simulink model "intrari_necunoscute"  (R2022b)
settings: Solver=VariableStepAuto  StartTime=0.0  StopTime=100  RelTol=1e-3
values from neighbouring files (symbols this model uses):
  A = [0 0 1 0 ... (first row only)    [cmsd_script.m]
  Ae = [A,E;zeros(1,5)]    [cmsd_script.m]
  B = [0,0 ... (first row only)    [cmsd_script.m]
  Be = [B; 0 0]    [cmsd_script.m]
  C = [1 0 0 0 ... (first row only)    [cmsd_script.m]
  Ce = [C ,zeros(2,1)]    [cmsd_script.m]
  E = [7 2 1 3]'    [cmsd_script.m]
  F = T*A-K1*C    [cmsd_script.m]
  H = E*pinv(C*E)    [cmsd_script.m]
  Ks = K1+K2    [cmsd_script.m]
  Le = place(Ae',Ce',[-5 -6 -7 -8 -9])'    [cmsd_script.m]
  T = eye(4)-H*C    [cmsd_script.m]
settings Model: Creator=Alex  LastModifiedBy=Alex

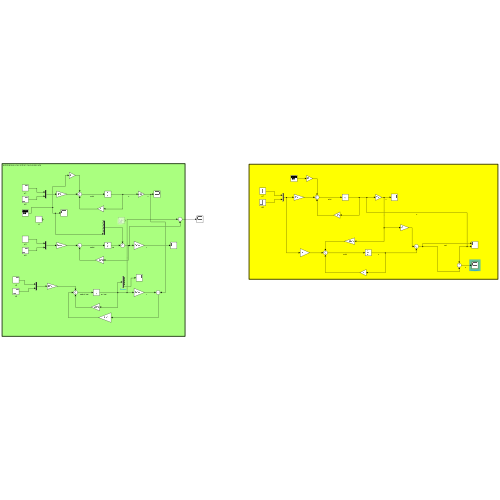
[thumbnail: Simulink's stored preview of the top-level diagram]
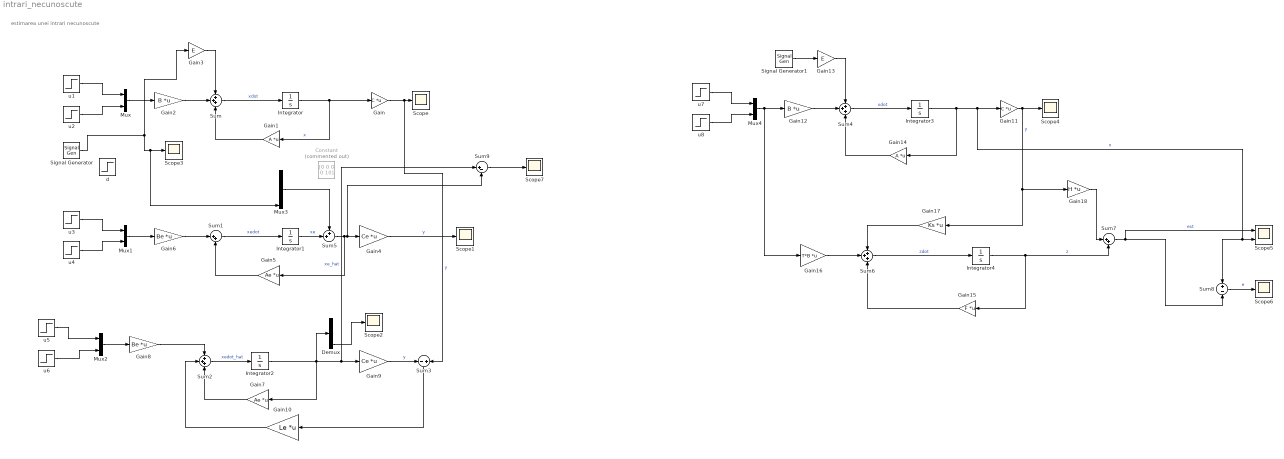
== system intrari_necunoscute ==
  note: estimarea unei intrari necunoscute
  Constant : Constant  Commented=on  Value=[0 0 0 0 10]
  Demux : Demux  Outputs=5
  Gain : Gain  Gain=C  Multiplication=Matrix(K*u)
  Gain1 : Gain  Gain=A  Multiplication=Matrix(K*u)
  Gain10 : Gain  Gain=Le  Multiplication=Matrix(K*u)
  Gain11 : Gain  Gain=C  Multiplication=Matrix(K*u)
  Gain12 : Gain  Gain=B  Multiplication=Matrix(K*u)
  Gain13 : Gain  Gain=E
  Gain14 : Gain  Gain=A  Multiplication=Matrix(K*u)
  Gain15 : Gain  Gain=F  Multiplication=Matrix(K*u)
  Gain16 : Gain  Gain=T*B  Multiplication=Matrix(K*u)
  Gain17 : Gain  Gain=Ks  Multiplication=Matrix(K*u)
  Gain18 : Gain  Gain=H  Multiplication=Matrix(K*u)
  Gain2 : Gain  Gain=B  Multiplication=Matrix(K*u)
  Gain3 : Gain  Gain=E
  Gain4 : Gain  Gain=Ce  Multiplication=Matrix(K*u)
  Gain5 : Gain  Gain=Ae  Multiplication=Matrix(K*u)
  Gain6 : Gain  Gain=Be  Multiplication=Matrix(K*u)
  Gain7 : Gain  Gain=Ae  Multiplication=Matrix(K*u)
  Gain8 : Gain  Gain=Be  Multiplication=Matrix(K*u)
  Gain9 : Gain  Gain=Ce  Multiplication=Matrix(K*u)
  Integrator{,1..4} (5 alike) : Integrator
  Mux{,1..2,4} (4 alike) : Mux  Inputs=2
  Mux3 : Mux  Inputs=5
  Scope{,1..4,6..7} (7 alike) : Scope
  Scope5 : Scope  NumInputPorts=2
  Signal Generator : SignalGenerator  WaveForm=square  Frequency=0.1
  Signal Generator1 : SignalGenerator
  Sum{,2,4,6} (4 alike) : Sum  Inputs=+++
  Sum1 : Sum  Inputs=|++
  Sum3 : Sum  Inputs=-+
  Sum5 : Sum  Inputs=++|
  Sum7 : Sum  Inputs=|++
  Sum8 : Sum  Inputs=+-
  Sum9 : Sum  Inputs=|+-
  d : Step  Time=0  After=10  SampleTime=0
  u{1,3,5,7} (4 alike) : Step  Time=0  After=0.1  SampleTime=0
  u{2,4,6,8} (4 alike) : Step  Time=0  After=0  SampleTime=0
  wires:
  Sum/1 -> Integrator/1  "xdot"
  Integrator/1 -> Gain/1, Gain1/1  "x"
  Gain/1 -> Sum3/2, Scope/1  "y"
  Gain2/1 -> Sum/2
  Gain3/1 -> Sum/1
  u1/1 -> Mux/1
  u2/1 -> Mux/2
  Mux/1 -> Gain2/1
  Gain1/1 -> Sum/3
  Gain5/1 -> Sum1/2
  Mux1/1 -> Gain6/1
  u4/1 -> Mux1/2
  u3/1 -> Mux1/1
  Sum1/1 -> Integrator1/1  "xedot"
  Gain6/1 -> Sum1/1
  Gain8/1 -> Sum2/1
  Sum2/1 -> Integrator2/1  "xedot_hat"
  Integrator2/1 -> Sum9/1, Gain9/1, Demux/1, Gain7/1  "xe_hat"
  u5/1 -> Mux2/1
  u6/1 -> Mux2/2
  Mux2/1 -> Gain8/1
  Gain9/1 -> Sum3/1  "y"
  Sum3/1 -> Gain10/1
  Gain7/1 -> Sum2/3
  Gain10/1 -> Sum2/2
  Demux/5 -> Scope2/1
  Integrator1/1 -> Sum5/2  "xe"
  Sum5/1 -> Sum9/2, Gain4/1, Gain5/1
  Signal Generator/1 -> Mux3/5, Scope3/1, Gain3/1
  Mux3/1 -> Sum5/1
  Mux4/1 -> Gain16/1, Gain12/1
  u8/1 -> Mux4/2
  u7/1 -> Mux4/1
  Gain13/1 -> Sum4/1
  Gain12/1 -> Sum4/2
  Gain11/1 -> Gain17/1, Gain18/1, Scope4/1  "y"
  Sum4/1 -> Integrator3/1  "xdot"
  Signal Generator1/1 -> Gain13/1
  Gain14/1 -> Sum4/3
  Integrator3/1 -> Gain14/1, Sum8/1, Scope5/2, Gain11/1  "x"
  Integrator4/1 -> Sum7/2, Gain15/1  "z"
  Sum6/1 -> Integrator4/1  "zdot"
  Gain15/1 -> Sum6/3
  Gain16/1 -> Sum6/2
  Gain17/1 -> Sum6/1
  Gain18/1 -> Sum7/1
  Sum7/1 -> Sum8/2, Scope5/1  "est"
  Sum8/1 -> Scope6/1  "e"
  Sum9/1 -> Scope7/1
  Gain4/1 -> Scope1/1  "y"
